simulink model "prob4"  (R2020b)
settings: Solver=VariableStepAuto  StartTime=0.0  StopTime=10.0  RelTol=1e-3
PostLoadFcn:
  | b0=1;
  | b1=0.4;
  | a0=0.5;
  | a1=0.25;
model workspace (MAT data in the model file):
  a0 = Simulink.Parameter
  a0.Value = 0.5
  a0.DataType = 'auto'
  a0.Dimensions = [1 1]
  a1 = Simulink.Parameter
  a1.Value = 0.25
  a1.DataType = 'auto'
  a1.Dimensions = [1 1]
  b0 = Simulink.Parameter
  b0.Value = 1
  b0.DataType = 'auto'
  b0.Dimensions = [1 1]
  b1 = Simulink.Parameter
  b1.Value = 0.4
  b1.DataType = 'auto'
  b1.Dimensions = [1 1]
settings Model: Creator=AVM  LastModifiedBy=AVM

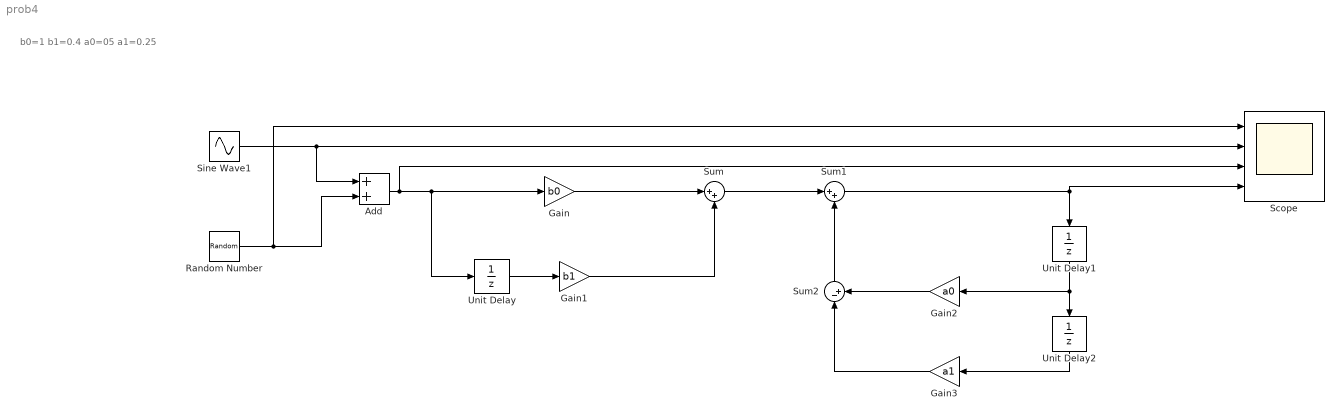
== system prob4 ==
  note: b0=1
      | b1=0.4
      | a0=05
      | a1=0.25
  Add : Sum
  Gain : Gain  Gain=b0
  Gain1 : Gain  Gain=b1
  Gain2 : Gain  Gain=a0
  Gain3 : Gain  Gain=a1
  Random Number : RandomNumber  SampleTime=0.1
  Scope : Scope  NumInputPorts=4
  Sine Wave1 : Sin  Amplitude=50  SampleTime=0
  Sum : Sum  Inputs=|++
  Sum1 : Sum  Inputs=|++
  Sum2 : Sum  Inputs=|-+
  Unit Delay : UnitDelay  SampleTime=-1  HasFrameUpgradeWarning=on
  Unit Delay1 : UnitDelay  SampleTime=-1  HasFrameUpgradeWarning=on
  Unit Delay2 : UnitDelay  SampleTime=-1  HasFrameUpgradeWarning=on
  wires:
  Gain2/1 -> Sum2/2
  Sine Wave1/1 -> Scope/2, Add/1
  Sum2/1 -> Sum1/2
  Gain3/1 -> Sum2/1
  Gain/1 -> Sum/1
  Unit Delay2/1 -> Gain3/1
  Unit Delay/1 -> Gain1/1
  Sum1/1 -> Unit Delay1/1, Scope/4
  Gain1/1 -> Sum/2
  Sum/1 -> Sum1/1
  Random Number/1 -> Scope/1, Add/2
  Unit Delay1/1 -> Gain2/1, Unit Delay2/1
  Add/1 -> Scope/3, Unit Delay/1, Gain/1
